simulink model "lab2"  (R2017b)
settings: Solver=ode4  StartTime=0.0  StopTime=10.0  FixedStep=0.01  RelTol=1e-3
libraries: simulink x2
settings Model: Creator=niquit  LastModifiedBy=niquit

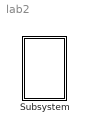
== system lab2 ==
  Subsystem : Subsystem  mask{G=9.81, M=100, x0=0, vx0=15, y0=5, vy0=0, R=2}

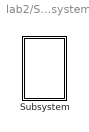
== system lab2/Subsystem ==
  Subsystem : Subsystem  mask{G=9.81, M=100, x0=0, y0=5, vx0=10, yx0=0, R=2}

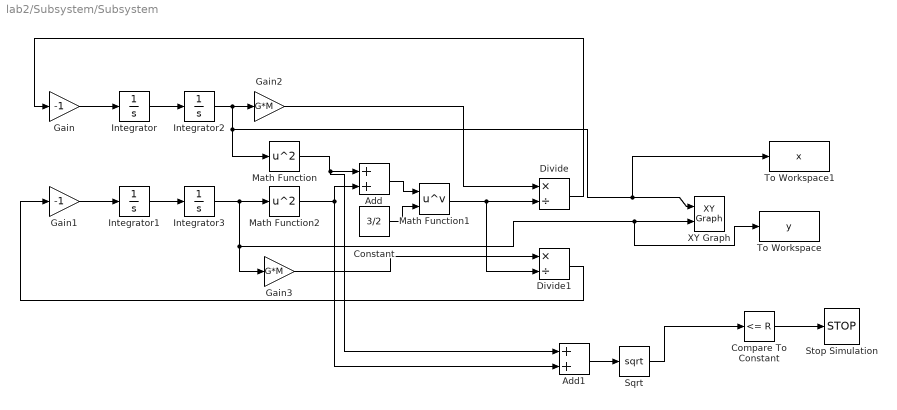
== system lab2/Subsystem/Subsystem ==
  Add : Sum
  Add1 : Sum
  Compare To Constant : simulink/Logic and Bit Operations/Compare To Constant  relop=<=  const=R  OutDataTypeStr=boolean
  Constant : Constant  Value=3/2
  Divide : Product  Inputs=*/
  Divide1 : Product  Inputs=*/
  Gain : Gain  Gain=-1
  Gain1 : Gain  Gain=-1
  Gain2 : Gain  Gain=G*M
  Gain3 : Gain  Gain=G*M
  Integrator : Integrator  InitialCondition=vx0
  Integrator1 : Integrator  InitialCondition=vy0
  Integrator2 : Integrator  InitialCondition=x0
  Integrator3 : Integrator  InitialCondition=y0
  Math Function : Math  Operator=square  SaturateOnIntegerOverflow=on
  Math Function1 : Math  Operator=pow  SaturateOnIntegerOverflow=on
  Math Function2 : Math  Operator=square  SaturateOnIntegerOverflow=on
  Sqrt : Sqrt  SaturateOnIntegerOverflow=on
  Stop Simulation : Stop
  To Workspace : ToWorkspace  VariableName=y  SampleTime=-1
  To Workspace1 : ToWorkspace  VariableName=x  SampleTime=-1
  XY Graph : simulink/Sinks/XY Graph  xmin=-10  xmax=10  ymin=-10  ymax=10  st=-1
  wires:
  Math Function2/1 -> Add1/2, Add/2
  Math Function1/1 -> Divide1/2, Divide/2
  Math Function/1 -> Add1/1, Add/1
  Integrator1/1 -> Integrator3/1
  Gain1/1 -> Integrator1/1
  Integrator/1 -> Integrator2/1
  Gain/1 -> Integrator/1
  Constant/1 -> Math Function1/2
  Compare To Constant/1 -> Stop Simulation/1
  Add1/1 -> Sqrt/1
  Divide/1 -> Gain/1
  Integrator3/1 -> Math Function2/1, Gain3/1, To Workspace/1, XY Graph/2
  Gain2/1 -> Divide/1
  Gain3/1 -> Divide1/1
  Divide1/1 -> Gain1/1
  Add/1 -> Math Function1/1
  Sqrt/1 -> Compare To Constant/1
  Integrator2/1 -> To Workspace1/1, XY Graph/1, Math Function/1, Gain2/1
